simulink model "test"  (R2016a)
settings: Solver=FixedStepAuto  StartTime=0.0  StopTime=10.0  FixedStep=0.1  RelTol=1e-3
undefined symbols (not defined in the file): sigbuilder_block
libraries: fuzblock x2
settings Model: Creator=Admin  LastModifiedBy=Admin

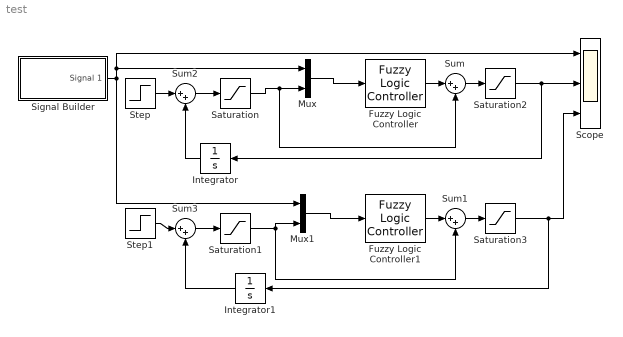
== system test ==
  Fuzzy Logic Controller : fuzblock/Fuzzy Logic  Controller  fis='left.fis'
  Fuzzy Logic Controller1 : fuzblock/Fuzzy Logic  Controller  fis='right.fis'
  Integrator : Integrator
  Integrator1 : Integrator
  Mux : Mux  Inputs=2
  Mux1 : Mux  Inputs=2
  Saturation{,1..3} (4 alike) : Saturate  UpperLimit=100  LowerLimit=-100
  Scope : Scope  NumInputPorts=3
  Signal Builder : Subsystem  Tag=STV Subsys  LoadFcn=sigbuilder_block('load',[404 117.5 550.5 362.5 ]);  StartFcn=sigbuilder_block('start');  StopFcn=sigbuilder_block('stop');  ClipboardFcn=sigbuilder_block('clipboard');  mask(Sigbuilder block){}
      mask help: Simulink:masks:SigbuilderBlock_MD
      mask init:
      | if ~strcmp(get_param(bdroot(gcbh),'SimulationStatus'),'stopped') tuvar = sigbuilder_block('maskInit'); end
      settings: CopyFcn=sigbuilder_block('copy');  DeleteFcn=sigbuilder_block('delete');  ModelCloseFcn=sigbuilder_block('modelClose');  PreSaveFcn=sigbuilder_block('preSave');  PauseFcn=sigbuilder_block('pause');  ContinueFcn=sigbuilder_block('continue');  NameChangeFcn=sigbuilder_block('namechange');  OpenFcn=sigbuilder_block('open',[404 117.5 550.5 362.5 ]);  CloseFcn=sigbuilder_block('close');
      mask Display: plot(0, 0, 100, 100,[2, 2, 32, 32, 2], [68, 8, 8, 68, 68],[32, 2], [38, 38], [32, 19, 2],[53, 60, 44], [32, 17, 17, 2],[16, 16, 31, 31]);txt = getActiveGroup(gcbh);text(2, 100, txt,'verticalAlignment', 'top');
  Step : Step  Before=50  After=0  SampleTime=0
  Step1 : Step  Before=50  After=0  SampleTime=0
  Sum{,1..3} (4 alike) : Sum  Inputs=|++
  wires:
  Signal Builder/1(Signal 1) -> Scope/1, Mux/1, Mux1/1
  Mux/1 -> Fuzzy Logic Controller/1
  Mux1/1 -> Fuzzy Logic Controller1/1
  Fuzzy Logic Controller/1 -> Sum/1
  Fuzzy Logic Controller1/1 -> Sum1/1
  Sum/1 -> Saturation2/1
  Sum1/1 -> Saturation3/1
  Sum3/1 -> Saturation1/1
  Sum2/1 -> Saturation/1
  Step/1 -> Sum2/1
  Step1/1 -> Sum3/1
  Integrator/1 -> Sum2/2
  Integrator1/1 -> Sum3/2
  Saturation/1 -> Sum/2, Mux/2
  Saturation1/1 -> Mux1/2, Sum1/2
  Saturation2/1 -> Integrator/1, Scope/2
  Saturation3/1 -> Integrator1/1, Scope/3

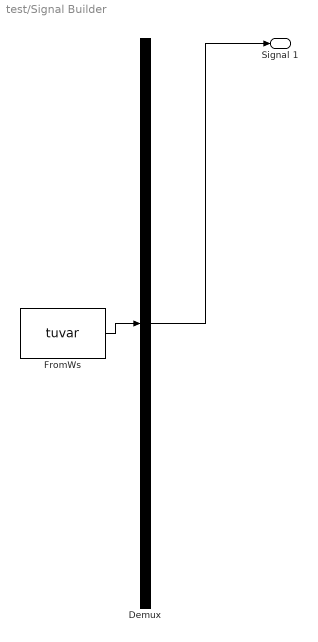
== system test/Signal Builder ==
  Demux : Demux  Tag=STV Demux  Outputs=1
  FromWs : FromWorkspace  Tag=STV FromWs  VariableName=tuvar  SampleTime=0
      SigBuilderData=|
      | common.afterFinalStr = 'Extrapolate'
      | common.sampleTime = 0
      | dataSet.timeRange = [0 10]
      | dataSet.name = 'Group 1'
      | sbobj.Groups.Name = 'Group 1'
      | sbobj.Groups.Signals.Name = 'Signal 1'
      | sbobj.Groups.Signals.XData = [0 1 1 4 4 6 6 8 8 10]
      | sbobj.Groups.Signals.YData = [0.5 0.5 -60 -60 29.5 29.5 0.5 0.5 -20.5 -20.5]
  Signal 1 : Outport  Tag=STV Outport
  wires:
  Demux/1 -> Signal 1/1
  FromWs/1 -> Demux/1
